simulink model "EOM_solver_cleaned"  (R2023b)
settings: Solver=ode45  StartTime=0.0  StopTime=1  RelTol=1e-3
values from neighbouring files (symbols this model uses):
  flow = [a_c;b_c;speed_c]    [EOM_input.m]
  M = M_a + M_rb    [EOM_input.m]    (also in Mechatronics (1).m; Mechatronics.m)
  tau = [tau_u;tau_v;tau_r]    [EOM_input.m]    (also in Mechatronics (1).m; Mechatronics.m)
  tau_e = [0; 0; 0]    [EOM_input.m]    (also in Mechatronics (1).m = 0; Mechatronics.m = [0 0 0])
settings Model: Creator=helle  LastModifiedBy=helle

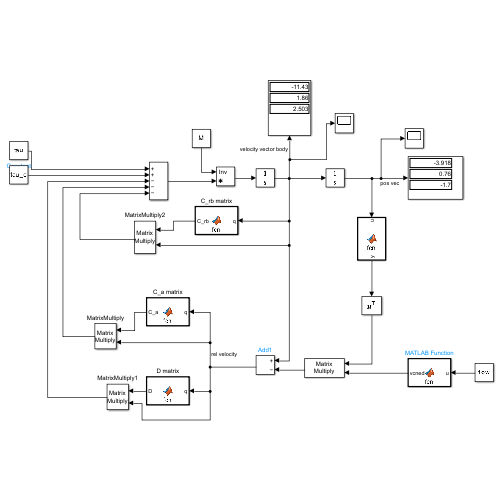
[thumbnail: Simulink's stored preview of the top-level diagram]
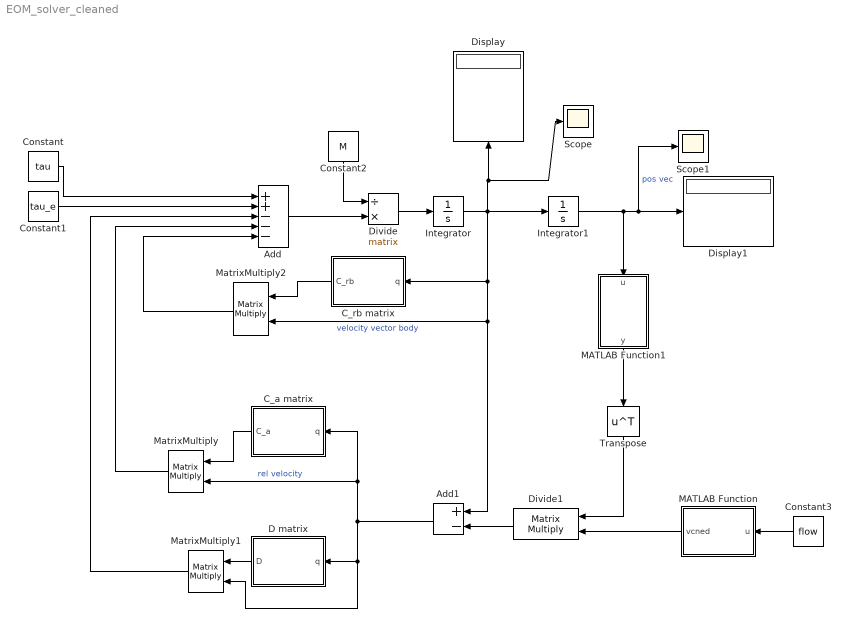
== system EOM_solver_cleaned ==
  Add : Sum  Inputs=++---
  Add1 : Sum  Inputs=+-
  C_a matrix : MATLAB Function  TreatAsAtomicUnit=on
  C_rb matrix : MATLAB Function  TreatAsAtomicUnit=on
  Constant : Constant  Value=tau
  Constant1 : Constant  Value=tau_e
  Constant2 : Constant  Value=M
  Constant3 : Constant  Value=flow
  D matrix : MATLAB Function  TreatAsAtomicUnit=on
  Display : Display
  Display1 : Display
  Divide : Product  Inputs=/*  Multiplication=Matrix(*)
  Divide1 : Product  Inputs=**  Multiplication=Matrix(*)
  Integrator : Integrator
  Integrator1 : Integrator
  MATLAB Function : MATLAB Function  TreatAsAtomicUnit=on
  MATLAB Function1 : MATLAB Function  TreatAsAtomicUnit=on
  MatrixMultiply : Product  Multiplication=Matrix(*)
  MatrixMultiply1 : Product  Multiplication=Matrix(*)
  MatrixMultiply2 : Product  Multiplication=Matrix(*)
  Scope : Scope
  Scope1 : Scope
  Transpose : Math  Operator=transpose
  wires:
  Constant/1 -> Add/1
  Constant1/1 -> Add/2
  Add/1 -> Divide/2
  Constant2/1 -> Divide/1
  Divide/1 -> Integrator/1
  Integrator/1 -> Integrator1/1, Scope/1, Display/1, Add1/1, MatrixMultiply2/2, C_rb matrix/1(q)  "velocity vector body"
  Integrator1/1 -> MATLAB Function1/1(u), Scope1/1, Display1/1  "pos vec"
  Constant3/1 -> MATLAB Function/1(u)
  MATLAB Function1/1(y) -> Transpose/1
  Transpose/1 -> Divide1/1
  MATLAB Function/1(vcned) -> Divide1/2
  Divide1/1 -> Add1/2
  Add1/1 -> MatrixMultiply1/2, D matrix/1(q), MatrixMultiply/2, C_a matrix/1(q)  "rel velocity"
  C_a matrix/1(C_a) -> MatrixMultiply/1
  D matrix/1(D) -> MatrixMultiply1/1
  MatrixMultiply/1 -> Add/4
  MatrixMultiply1/1 -> Add/3
  C_rb matrix/1(C_rb) -> MatrixMultiply2/1
  MatrixMultiply2/1 -> Add/5

== matlab function EOM_solver_cleaned/MATLAB Function ==
  data: u input; vcned output
function vcned = fcn(u)
a=u(1);
b=u(2);
c=u(3);
vcned=[c*cos(a)*cos(b) ;c*sin(b); c*sin(a)*cos(b)];

== matlab function EOM_solver_cleaned/C_a matrix ==
  data: q input; C_a output
function C_a = fcn(q)
u = q(1);
v = q(2);
r = q(3);

w = 0; % heave
p = 0; % roll
q = 0; % pitch

X_dotu = 1.2; % all of this given
X_dotv = 0;
X_dotw = 0;
X_dotp = 0;
X_dotq = 0;
X_dotr = 0;

Y_dotu = 0; 
Y_dotv = 66.1; 
Y_dotw = 0;
Y_dotp = 0;
Y_dotq = 0;
Y_dotr = 0;

a_1 = X_dotu*u + X_dotv*v +X_dotw*w + X_dotp*p + X_dotq*q +X_dotr*r;
a_2 = Y_dotu*u + Y_dotv*v +Y_dotw*w + Y_dotp*p + Y_dotq*q +Y_dotr*r;

C_a = [0,   0,   a_2;
       0,   0,  -a_1;
      -a_2, a_1,  0];

== matlab function EOM_solver_cleaned/D matrix ==
  data: q input; D output
function D = fcn(q)
u = q(1);
v = q(2);
r = q(3);

d_11 = 0.0069*u^3 - 0.1314*u^2 + 0.8842*u - 2.0431;  %X_drag
d_22 = 0.0289*v^3 - 0.5191*v^2 + 3.3058*v - 2.3601;  %Y_drag
c1 = 122.3;
c2 = 4.8;
L = 0.97;
d_33 = (1/80)*c1*r^3*L^4 + (1/12)*c2*r*L^2;

D = [d_11, 0,   0;
      0,  d_22, 0;
      0,   0,  d_33];

== matlab function EOM_solver_cleaned/C_rb matrix ==
  data: q input; C_rb output
function C_rb = fcn(q)
u = q(1);
v = q(2);
r = q(3);

x_g = 0; % body fixed reference system located at COG
y_g = 0;
m = 18; % Mass

C_rb = [0,0, -m*(x_g*r+v);
        0,0, -m*(y_g*r-u);
        m*(x_g*r + v), m*(y_g*r- u),0];

== matlab function EOM_solver_cleaned/MATLAB Function1 ==
  data: u input; y output
function y = fcn(u)
psi=u(3);

y = [cos(psi),-sin(psi),0;
    sin(psi),cos(psi),0;
    0,0,1];
